simulink model "v0_VoltageImitator_ramp_generator"  (R2020b)
settings: Solver=ode23t  StartTime=0.0  StopTime=1  RelTol=1e-3
libraries: powerlib x10, powerlib_meascontrol x1
settings Model: Creator=Александр  LastModifiedBy=Александр

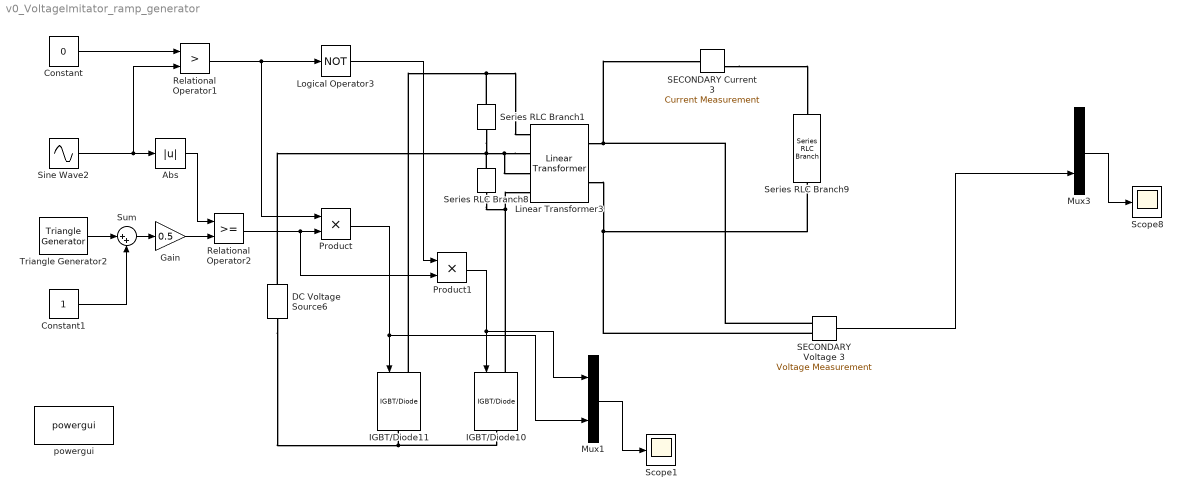
== system v0_VoltageImitator_ramp_generator ==
  Abs : Abs
  Constant : Constant  Value=0
  Constant1 : Constant
  DC Voltage Source6 : powerlib/Electrical Sources/DC Voltage Source  Amplitude=12  Measurements=None
  Gain : Gain  Gain=0.5
  IGBT/Diode10 : powerlib/Power Electronics/IGBT//Diode  Ron=1e-3  Rs=1e5  Cs=inf  Measurements=off
  IGBT/Diode11 : powerlib/Power Electronics/IGBT//Diode  Ron=1e-3  Rs=1e5  Cs=inf  Measurements=off
  Linear Transformer3 : powerlib/Elements/Linear Transformer  UNITS=SI  NominalPower=[ 10000 50 ]  winding1=[220 2950 2.2]  winding2=[12 43.2 10.4e-3]  ThreeWindings=on  winding3=[12 43.2 10.4e-3]  RmLm=[4444 24.3]  Measurements=None  DataType=on
  Logical Operator3 : Logic  Operator=NOT  IconShape=distinctive  AllPortsSameDT=off  OutDataTypeStr=boolean
  Mux1 : Mux  Inputs=2
  Mux3 : Mux  Inputs=2
  Product : Product
  Product1 : Product
  Relational Operator1 : RelationalOperator  Operator=>  OutDataTypeStr=boolean  RndMeth=Nearest
  Relational Operator2 : RelationalOperator  OutDataTypeStr=boolean  RndMeth=Nearest
  SECONDARY Current 3 : powerlib/Measurements/Current Measurement  PhasorSimulation=off  OutputType=Complex  PSBequivalent=0
  SECONDARY Voltage 3 : powerlib/Measurements/Voltage Measurement  PhasorSimulation=off  OutputType=Complex  PSBequivalent=0
  Scope1 : Scope
  Scope8 : Scope
  Series RLC Branch1 : powerlib/Elements/Series RLC Branch  LConnTagsString=__new0  RConnTagsString=__new0  BranchType=RC  Resistance=10  Inductance=50e-3  SetiL0=off  InitialCurrent=0  Capacitance=1e-6  Setx0=off  InitialVoltage=0  Measurements=None
  Series RLC Branch8 : powerlib/Elements/Series RLC Branch  LConnTagsString=__new0  RConnTagsString=__new0  BranchType=RC  Resistance=10  Inductance=50e-3  SetiL0=off  InitialCurrent=0  Capacitance=1e-6  Setx0=off  InitialVoltage=0  Measurements=None
  Series RLC Branch9 : powerlib/Elements/Series RLC Branch  LConnTagsString=__new0  RConnTagsString=__new0  BranchType=R  Resistance=100000  Inductance=1e-3  SetiL0=off  InitialCurrent=0  Capacitance=1e-6  Setx0=off  InitialVoltage=0  Measurements=None
  Sine Wave2 : Sin  Frequency=2*pi*50  SampleTime=0
  Sum : Sum  Inputs=|++
  Triangle Generator2 : powerlib_meascontrol/Pulse & Signal Generators/Triangle Generator  Freq=10000  Phase=90  Ts=0
  powergui : powerlib/powergui  Priority=1  SimulationMode=Continuous  SampleTime=50e-6  frequency=60  Iterations=50  frequencyindice=0  Pbase=100e6  ErrMax=1e-4  UnitsV=kV  UnitsW=MW  buscounter=0  FunctionMessages=off  echomessages=off  EnableUseOfTLC=off  CurrentSourceSwitches=off  DisableSnubberDevices=off  DisableRonSwitches=off  DisableVfSwitches=off  DisplayEquations=off  AutomaticDiscreteSolvers=off  SolverType=Tustin/Backward Euler (TBE)  Interpol=off  ExternalGateDelay=off  methode=off  Ts=100  x0status=blocks  SPID=on  SwTol=0  HookPort=off  NonlinearTolerance=1e-4  nMaxIteration=100  ContinueOnMaxIteration=off  RestoreLinks=warning  ResistiveCurrentMeasurement=off  Frange=[0:2:500]  Ylog=off  Xlog=on  ShowGrid=off  save=off  variable=ZData  structure=0  ZoomFFT=off  StartTime=0.0  cycles=1  DisplayStyle=1  fundamental=60  FreqAxis=off  MaxFrequency=1000  frequencyindicesteady=1  RmsSteady=1  display=off
  wires:
  Mux3/1 -> Scope8/1
  Constant/1 -> Relational Operator1/1
  Sine Wave2/1 -> Abs/1, Relational Operator1/2
  Relational Operator2/1 -> Product1/2, Product/2
  Relational Operator1/1 -> Product/1, Logical Operator3/1
  Product/1 -> Mux1/2, IGBT/Diode11/1
  Product1/1 -> Mux1/1, IGBT/Diode10/1
  Logical Operator3/1 -> Product1/1
  SECONDARY Voltage 3/1 -> Mux3/2
  Mux1/1 -> Scope1/1
  Abs/1 -> Relational Operator2/1
  Triangle Generator2/1 -> Sum/1
  Constant1/1 -> Sum/2
  Gain/1 -> Relational Operator2/2
  Sum/1 -> Gain/1
  connections:
  Linear Transformer3/LConn2 -- SECONDARY Voltage 3/LConn2 -- Series RLC Branch9/RConn1
  Linear Transformer3/RConn2 -- Series RLC Branch1/RConn1 -- Series RLC Branch8/LConn1 -- DC Voltage Source6/RConn1 -- Linear Transformer3/RConn3
  IGBT/Diode10/LConn1 -- Series RLC Branch8/RConn1 -- Linear Transformer3/RConn4
  Linear Transformer3/LConn1 -- SECONDARY Voltage 3/LConn1 -- SECONDARY Current 3/LConn1
  IGBT/Diode11/LConn1 -- Series RLC Branch1/LConn1 -- Linear Transformer3/RConn1
  SECONDARY Current 3/RConn1 -- Series RLC Branch9/LConn1
  IGBT/Diode10/RConn1 -- DC Voltage Source6/LConn1 -- IGBT/Diode11/RConn1
